simulink model "buck"  (R2019b)
settings: Solver=VariableStepAuto  StartTime=0.0  StopTime=3  RelTol=1e-3
values from neighbouring files (symbols this model uses):
  C = 46.67*10^(-9)    (= 4.667e-08)    [Parameters.m]
  L = 208.3*10^(-6)    (= 0.0002083)    [Parameters.m]
  R = 1.667    [Parameters.m]
  Vin = 12    [Parameters.m]
settings Model: Creator=60255  LastModifiedBy=60255

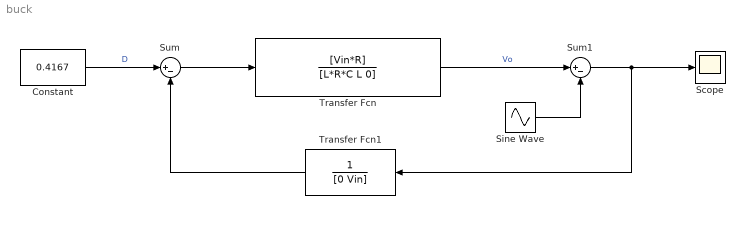
== system buck ==
  Constant : Constant  Value=0.4167
  Scope : Scope
  Sine Wave : Sin  Amplitude=0.5  Frequency=100  SampleTime=0
  Sum : Sum  Inputs=|+-
  Sum1 : Sum  Inputs=|+-
  Transfer Fcn : TransferFcn  Numerator=[Vin*R]  Denominator=[L*R*C L 0]
  Transfer Fcn1 : TransferFcn  Denominator=[0 Vin]
  wires:
  Sum/1 -> Transfer Fcn/1
  Constant/1 -> Sum/1  "D"
  Transfer Fcn1/1 -> Sum/2
  Transfer Fcn/1 -> Sum1/1  "Vo"
  Sine Wave/1 -> Sum1/2
  Sum1/1 -> Transfer Fcn1/1, Scope/1
